simulink model "Wtg"  (R2018b)
settings: Solver=VariableStepAuto  StartTime=0.0  StopTime=10.0  RelTol=1e-3
values from neighbouring files (symbols this model uses):
  beta = 0    [ini_wtg.m]
  C_1 = 0.73    [ini_wtg.m]
  C_2 = 151    [ini_wtg.m]
  C_3 = 0.58    [ini_wtg.m]
  C_4 = 13.2    [ini_wtg.m]
  C_5 = 18.4    [ini_wtg.m]
  C_7 = 0.002    [ini_wtg.m]
  C_8 = 2.14    [ini_wtg.m]
  lambda = 7.2    [ini_wtg.m]
  n_b = 0.95    [ini_wtg.m]
  n_g = 0.97    [ini_wtg.m]
  radio = 42    [ini_wtg.m]
  ro = 1.225    [ini_wtg.m]
settings Model: Creator=Pedro  LastModifiedBy=Pedro

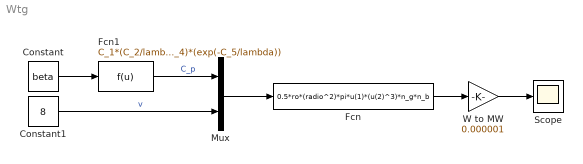
== system Wtg ==
  Constant : Constant  Value=beta
  Constant1 : Constant  Value=8
  Fcn : Fcn  Expr=0.5*ro*(radio^2)*pi*u(1)*(u(2)^3)*n_g*n_b
  Fcn1 : Fcn  Expr=C_1*(C_2/lambda-C_3*u(1)-C_7*u(1)^C_8-C_4)*(exp(-C_5/lambda))
  Mux : Mux  Inputs=2
  Scope : Scope
  W to MW : Gain  Gain=0.000001
  wires:
  Mux/1 -> Fcn/1
  Fcn1/1 -> Mux/1  "C_p"
  Constant1/1 -> Mux/2  "v"
  Constant/1 -> Fcn1/1
  Fcn/1 -> W to MW/1
  W to MW/1 -> Scope/1
